simulink model "e02 1"  (R2023a)
settings: Solver=VariableStepAuto  StartTime=0.0  StopTime=6  RelTol=1e-3
values from neighbouring files (symbols this model uses):
  a0 = double(sol.a0)    [Grp43_part2_code.m]    (also in e01 2.m = double(S.a0); grp43_asgn2_2.m = double(S.a0))
  a1 = double(sol.a1)    [Grp43_part2_code.m]    (also in e01 2.m = double(S.a1); grp43_asgn2_2.m = double(S.a1))
  g = 9.8    [Grp43_Code.m]    (also in Grp43_part2_code.m = 9.81; e01 2.m; grp43_asgn2_2.m)
  l = 0.36    [Grp43_Code.m]    (also in Grp43_part2_code.m; e01 2.m; grp43_asgn2_2.m)
  m = 0.26    [Grp43_Code.m]    (also in Grp43_part2_code.m; e01 2.m; grp43_asgn2_2.m)
  M = 2.4    [Grp43_Code.m]    (also in Grp43_part2_code.m; e01 2.m; grp43_asgn2_2.m)
  p0 = double(sol.p0)    [Grp43_part2_code.m]    (also in e01 2.m = double(S.p0); grp43_asgn2_2.m = double(S.p0))
  p1 = double(sol.p1)    [Grp43_part2_code.m]    (also in e01 2.m = double(S.p1); grp43_asgn2_2.m = double(S.p1))
  q0 = double(sol.q0)    [Grp43_part2_code.m]    (also in e01 2.m = double(S.q0); grp43_asgn2_2.m = double(S.q0))
settings Model: Creator=jitbi  LastModifiedBy=jitbi

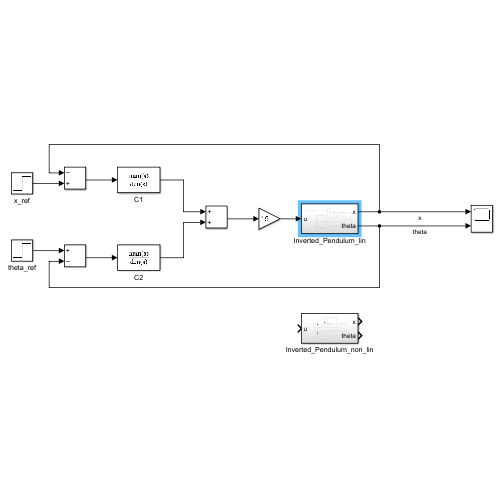
[thumbnail: Simulink's stored preview of the top-level diagram]
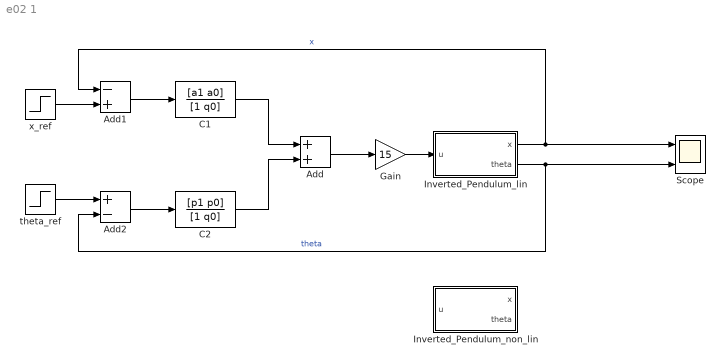
== system e02 1 ==
  Add : Sum
  Add1 : Sum  Inputs=-+
  Add2 : Sum  Inputs=+-
  C1 : TransferFcn  Numerator=[a1 a0]  Denominator=[1 q0]
  C2 : TransferFcn  Numerator=[p1 p0]  Denominator=[1 q0]
  Gain : Gain  Gain=15
  Inverted_Pendulum_lin : Subsystem
  Inverted_Pendulum_non_lin : Subsystem
  Scope : Scope  NumInputPorts=2
  theta_ref : Step  Time=0  SampleTime=1e-6
  x_ref : Step  Time=0  SampleTime=1e-6
  wires:
  C1/1 -> Add/1
  C2/1 -> Add/2
  x_ref/1 -> Add1/2
  Add1/1 -> C1/1
  theta_ref/1 -> Add2/1
  Add2/1 -> C2/1
  Add/1 -> Gain/1
  Inverted_Pendulum_lin/1(x) -> Scope/1, Add1/1  "x"
  Inverted_Pendulum_lin/2(theta) -> Add2/2, Scope/2  "theta"
  Gain/1 -> Inverted_Pendulum_lin/1(u)

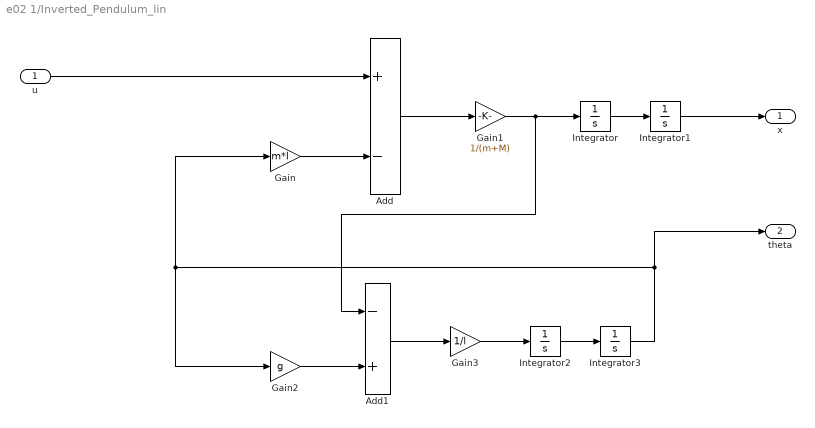
== system e02 1/Inverted_Pendulum_lin ==
  u : Inport
  Add : Sum  Inputs=+-
  Add1 : Sum  Inputs=-+
  Gain : Gain  Gain=m*l
  Gain1 : Gain  Gain=1/(m+M)
  Gain2 : Gain  Gain=g
  Gain3 : Gain  Gain=1/l
  Integrator{,1..3} (4 alike) : Integrator
  x : Outport
  theta : Outport  Port=2
  wires:
  u/1 -> Add/1
  Gain/1 -> Add/2
  Integrator3/1 -> theta/1, Gain/1, Gain2/1
  Add/1 -> Gain1/1
  Integrator/1 -> Integrator1/1
  Gain1/1 -> Add1/1, Integrator/1
  Integrator1/1 -> x/1
  Gain2/1 -> Add1/2
  Add1/1 -> Gain3/1
  Integrator2/1 -> Integrator3/1
  Gain3/1 -> Integrator2/1

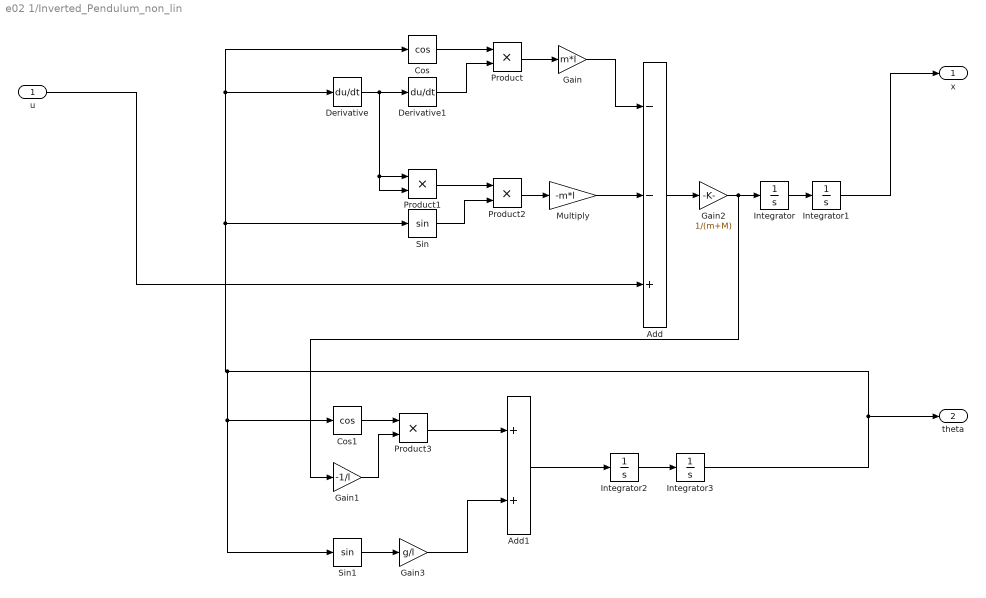
== system e02 1/Inverted_Pendulum_non_lin ==
  u : Inport
  Add : Sum  Inputs=--+
  Add1 : Sum
  Cos : Trigonometry  Operator=cos
  Cos1 : Trigonometry  Operator=cos
  Derivative : Derivative
  Derivative1 : Derivative
  Gain : Gain  Gain=m*l
  Gain1 : Gain  Gain=-1/l
  Gain2 : Gain  Gain=1/(m+M)
  Gain3 : Gain  Gain=g/l
  Integrator{,1..3} (4 alike) : Integrator
  Multiply : Gain  Gain=-m*l
  Product{,1..3} (4 alike) : Product
  Sin : Trigonometry
  Sin1 : Trigonometry
  x : Outport
  theta : Outport  Port=2
  wires:
  Product2/1 -> Multiply/1
  Integrator3/1 -> Cos1/1, Sin1/1, Cos/1, Derivative/1, Sin/1, theta/1
  Add/1 -> Gain2/1
  Cos/1 -> Product/1
  Derivative/1 -> Product1/1, Product1/2, Derivative1/1
  u/1 -> Add/3
  Derivative1/1 -> Product/2
  Product/1 -> Gain/1
  Multiply/1 -> Add/2
  Integrator/1 -> Integrator1/1
  Gain2/1 -> Gain1/1, Integrator/1
  Product1/1 -> Product2/1
  Sin/1 -> Product2/2
  Gain/1 -> Add/1
  Integrator1/1 -> x/1
  Cos1/1 -> Product3/1
  Gain1/1 -> Product3/2
  Sin1/1 -> Gain3/1
  Product3/1 -> Add1/1
  Gain3/1 -> Add1/2
  Add1/1 -> Integrator2/1
  Integrator2/1 -> Integrator3/1
